simulink model "magnetorquerCaracteristicas"  (R2024a)
settings: Solver=FixedStepAuto  StartTime=0.0  StopTime=tf  FixedStep=step_modelo  RelTol=1e-3
undefined symbols (not defined in the file or in its folder): sat_torquerod, TdTorq, TpulseTorq
settings Model: PacingRate=1000  VariantFading=off  Creator=rodri  LastModifiedBy=rodri
settings DataIOCC: SaveOutput=off  SaveTime=off
settings RTWCC: GPUComputeCapability=3.5

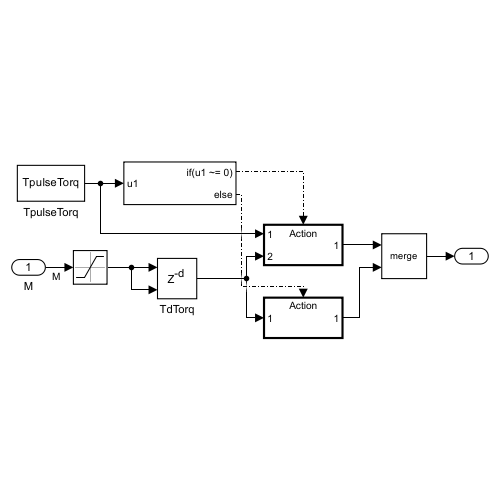
[thumbnail: Simulink's stored preview of the top-level diagram]
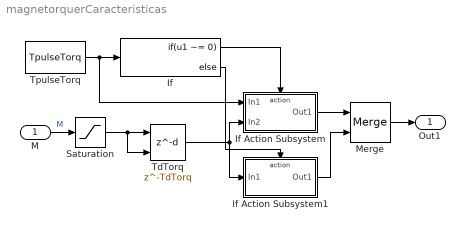
== system magnetorquerCaracteristicas ==
  M : Inport  OutDataTypeStr=double  PortDimensions=[1 1]  SampleTime=0
  If : If  IfExpression=u1 ~= 0
  If Action Subsystem : Subsystem  TreatAsAtomicUnit=on
  If Action Subsystem1 : Subsystem  TreatAsAtomicUnit=on
  Merge : Merge
  Saturation : Saturate  UpperLimit=sat_torquerod  LowerLimit=-sat_torquerod
  TdTorq : Delay  DelayLength=TdTorq  InitialConditionSource=Input port  InitialCondition=0
      settings: InputPortMap=u0,p4
  TpulseTorq : Constant  Value=TpulseTorq  SampleTime=-1
  Out1 : Outport  OutDataTypeStr=double  PortDimensions=[1 1]  SampleTime=0
  wires:
  M/1 -> Saturation/1  "M"
  If Action Subsystem/1(Out1) -> Merge/1
  If/1 -> If Action Subsystem/Action
  If/2 -> If Action Subsystem1/Action
  Saturation/1 -> TdTorq/2, TdTorq/1
  If Action Subsystem1/1(Out1) -> Merge/2
  TdTorq/1 -> If Action Subsystem/2(In2), If Action Subsystem1/1(In1)
  TpulseTorq/1 -> If/1, If Action Subsystem/1(In1)
  Merge/1 -> Out1/1

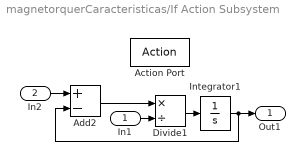
== system magnetorquerCaracteristicas/If Action Subsystem ==
  In1 : Inport
  In2 : Inport  Port=2
  Action Port : ActionPort
  Add2 : Sum  Inputs=+-
  Divide1 : Product  Inputs=*/
  Integrator1 : Integrator
  Out1 : Outport
  wires:
  In1/1 -> Divide1/2
  Divide1/1 -> Integrator1/1
  Add2/1 -> Divide1/1
  Integrator1/1 -> Out1/1, Add2/2
  In2/1 -> Add2/1

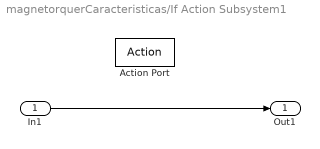
== system magnetorquerCaracteristicas/If Action Subsystem1 ==
  In1 : Inport
  Action Port : ActionPort
  Out1 : Outport
  wires:
  In1/1 -> Out1/1
